simulink model "lab4_simulink3model1"  (R2024a)
settings: Solver=VariableStepAuto  StartTime=0.0  StopTime=10.0  RelTol=1e-3
undefined symbols (not defined in the file or in its folder): DiscIntNeverNeededParam
libraries: commchan3 x1, dspfdesign x1, commanapbnd3 x1, dspsrcs4 x1
settings Model: Creator=pulley  LastModifiedBy=PULLEY

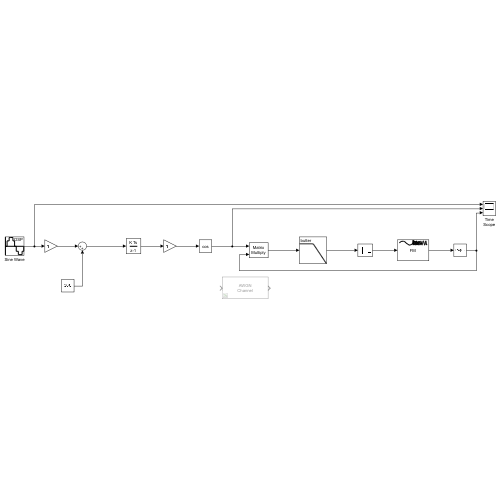
[thumbnail: Simulink's stored preview of the top-level diagram]
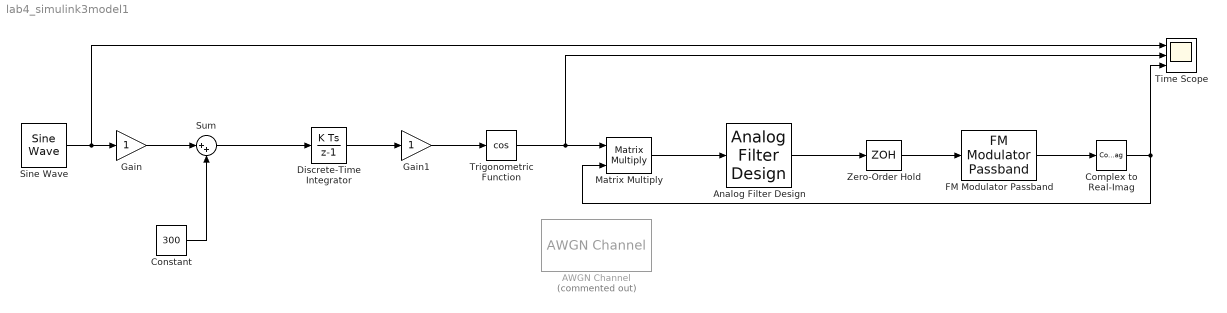
== system lab4_simulink3model1 ==
  AWGN Channel : commchan3/AWGN Channel  Commented=on  LegacyMode=off  NoiseMethod="Signal to noise ratio  (SNR)"  noiseMode="Signal to noise ratio  (SNR)"  EbNo=10  EsNo=10  SNR=10  BitsPerSymbol=1  SignalPower=1  SamplesPerSymbol=1  SymbolPeriod=1  VarianceSource=Parameter  Variance=1  RandomStream=Global stream  Seed=67  SimulateUsing=Code generation
  Analog Filter Design : dspfdesign/Analog Filter Design  method=Butterworth  filttype=Lowpass  N=10  Wlo=2*pi*10  Whi=80  Rp=2  Rs=40
  Complex to Real-Imag : ComplexToRealImag  Output=Real
  Constant : Constant  Value=300
  Discrete-Time Integrator : DiscreteIntegrator  SampleTime=1/98000  ICPrevOutput=DiscIntNeverNeededParam  ICPrevScaledInput=DiscIntNeverNeededParam
  FM Modulator Passband : commanapbnd3/FM Modulator Passband  Fc=10  Ph=0  Kc=50
  Gain : Gain
  Gain1 : Gain
  Matrix Multiply : Product  Multiplication=Matrix(*)
  Sine Wave : dspsrcs4/Sine Wave  Amplitude=1  Frequency=10  Phase=90  SampleMode=Discrete  OutComplex=Real  CompMethod=Trigonometric fcn  TableSize=Speed  SampleTime=1/98000  SamplesPerFrame=1  ResetState=Restart at time zero  OutputFrames=off  dataType=double  wordLen=16  udDataType=sfix(16)  fracBitsMode=Best precision  numFracBits=15  OutDataTypeStr=double  LastOutDataTypeStr=double
  Sum : Sum  Inputs=|++
  Time Scope : Scope  NumInputPorts=3
  Trigonometric Function : Trigonometry  Operator=cos
  Zero-Order Hold : ZeroOrderHold  SampleTime=-1
  wires:
  Sine Wave/1 -> Gain/1, Time Scope/1
  Gain/1 -> Sum/1
  Constant/1 -> Sum/2
  Sum/1 -> Discrete-Time Integrator/1
  Discrete-Time Integrator/1 -> Gain1/1
  Gain1/1 -> Trigonometric Function/1
  Trigonometric Function/1 -> Matrix Multiply/1, Time Scope/2
  Matrix Multiply/1 -> Analog Filter Design/1
  Analog Filter Design/1 -> Zero-Order Hold/1
  Zero-Order Hold/1 -> FM Modulator Passband/1
  FM Modulator Passband/1 -> Complex to Real-Imag/1
  Complex to Real-Imag/1 -> Time Scope/3, Matrix Multiply/2
